simulink model "casedevsnew"  (Simulink 7.9)
settings: Solver=ode45  StartTime=0.0  StopTime=10.0  RelTol=1e-3
undefined symbols (not defined in the file or in its folder): PreNode
libraries: Post_CommonlyUsedBlocks x18, Pre_CommonlyUsedBlocks x14
settings Model: Creator=jdenil  LastModifiedBy=jdenil

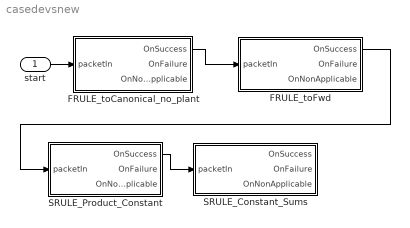
== system casedevsnew ==
  start : Inport
  FRULE_toCanonical_no_plant : Subsystem
  FRULE_toFwd : Subsystem
  SRULE_Constant_Sums : Subsystem
  SRULE_Product_Constant : Subsystem
  wires:
  start/1 -> FRULE_toCanonical_no_plant/1(packetIn)
  FRULE_toFwd/1(OnSuccess) -> SRULE_Product_Constant/1(packetIn)
  FRULE_toCanonical_no_plant/1(OnSuccess) -> FRULE_toFwd/1(packetIn)
  SRULE_Product_Constant/1(OnSuccess) -> SRULE_Constant_Sums/1(packetIn)

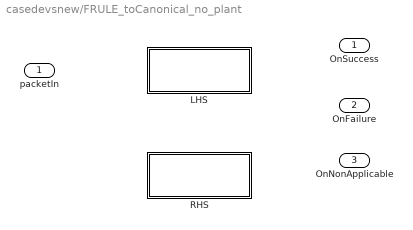
== system casedevsnew/FRULE_toCanonical_no_plant ==
  packetIn : Inport
  LHS : Subsystem  mask{Constraint=return True}
  RHS : Subsystem  mask{Action=[]}
  OnSuccess : Outport
  OnFailure : Outport  Port=2
  OnNonApplicable : Outport  Port=3

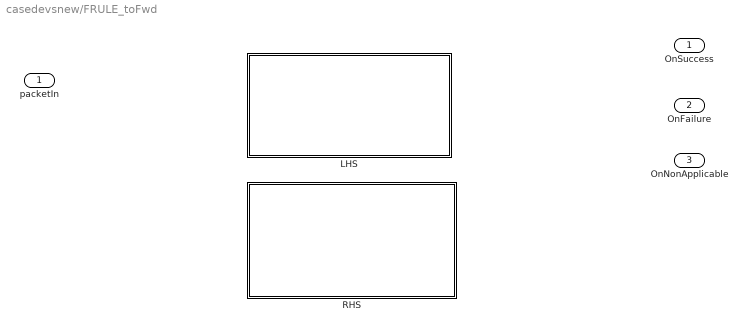
== system casedevsnew/FRULE_toFwd ==
  packetIn : Inport
  LHS : Subsystem
  RHS : Subsystem
  OnSuccess : Outport
  OnFailure : Outport  Port=2
  OnNonApplicable : Outport  Port=3

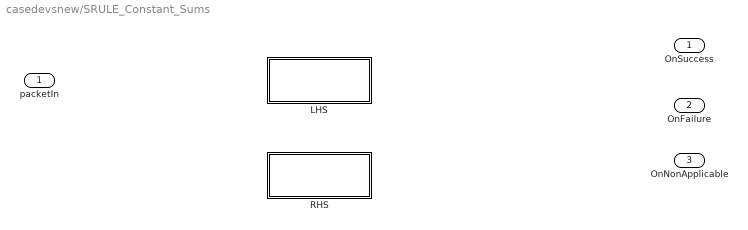
== system casedevsnew/SRULE_Constant_Sums ==
  packetIn : Inport
  LHS : Subsystem
  RHS : Subsystem
  OnSuccess : Outport
  OnFailure : Outport  Port=2
  OnNonApplicable : Outport  Port=3

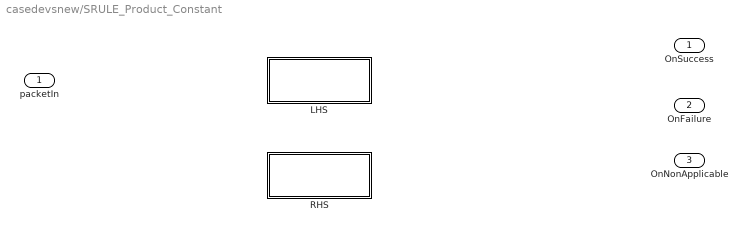
== system casedevsnew/SRULE_Product_Constant ==
  packetIn : Inport
  LHS : Subsystem
  RHS : Subsystem
  OnSuccess : Outport
  OnFailure : Outport  Port=2
  OnNonApplicable : Outport  Port=3

== system casedevsnew/FRULE_toCanonical_no_plant/LHS ==
  Atomic Subsystem : Subsystem  TreatAsAtomicUnit=on  mask{p_label=9, pre_Name=return False if 'plant' in attr_value else True, pre_Position=return True}
      settings: AttributesFormatString=%<p_label>

== system casedevsnew/FRULE_toCanonical_no_plant/RHS ==
  Atomic Subsystem : Subsystem  TreatAsAtomicUnit=on  mask{p_label=9, post_Name=return attr_value, post_Position=return attr_value}
      settings: AttributesFormatString=%<p_label>

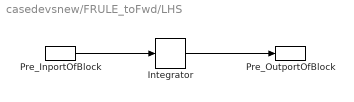
== system casedevsnew/FRULE_toFwd/LHS ==
  Integrator : Pre_CommonlyUsedBlocks/Integrator  pre_label=1  pre_initial=return True  pre_Name=return True  pre_Position=return True
      settings: AttributesFormatString=%<pre_label>
  Pre_InportOfBlock : Pre_CommonlyUsedBlocks/Pre_InportOfBlock  pre_label=0
      settings: AttributesFormatString=%<pre_label>
  Pre_OutportOfBlock : Pre_CommonlyUsedBlocks/Pre_OutportOfBlock  pre_label=2
      settings: AttributesFormatString=%<pre_label>
  wires:
  Pre_InportOfBlock/1 -> Integrator/1
  Integrator/1 -> Pre_OutportOfBlock/1

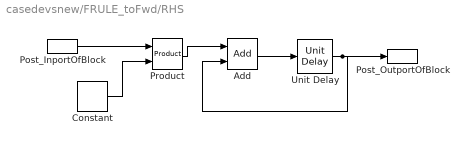
== system casedevsnew/FRULE_toFwd/RHS ==
  Add : Post_CommonlyUsedBlocks/Add  post_label=4  post_Name=return PreNode('1')['Name']+'Add'  post_Position=return PreNode('1')['Position']  post_Inputs=return '|++'
      settings: AttributesFormatString=%<post_label>
  Constant : Post_CommonlyUsedBlocks/Constant  post_label=6  post_value=return 0.001  post_Name=return PreNode('1')['Name']+'gainconst'  post_Position=return PreNode('1')['Position']
      settings: AttributesFormatString=%<post_label>
  Post_InportOfBlock : Post_CommonlyUsedBlocks/Post_InportOfBlock  post_label=0
      settings: AttributesFormatString=%<post_label>
  Post_OutportOfBlock : Post_CommonlyUsedBlocks/Post_OutportOfBlock  post_label=2
      settings: AttributesFormatString=%<post_label>
  Product : Post_CommonlyUsedBlocks/Product  post_label=3  post_Name=return PreNode('1')['Name']+'Product'  post_Position=return PreNode('1')['Position']
      settings: AttributesFormatString=%<post_label>
  Unit Delay : Post_CommonlyUsedBlocks/Unit Delay  post_label=5  post_initial=return PreNode('1')['InitialCondition']  post_Name=return PreNode('1')['Name']+'Delay'  post_Position=return PreNode('1')['Position']  post_SampleTime=return 0.001
      settings: AttributesFormatString=%<post_label>
  wires:
  Post_InportOfBlock/1 -> Product/1
  Product/1 -> Add/1
  Add/1 -> Unit Delay/1
  Unit Delay/1 -> Post_OutportOfBlock/1, Add/2
  Constant/1 -> Product/2

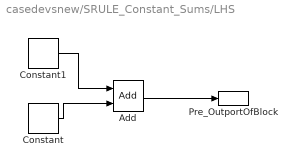
== system casedevsnew/SRULE_Constant_Sums/LHS ==
  Add : Pre_CommonlyUsedBlocks/Add  pre_label=0  pre_Name=return True  pre_Position=return True  pre_Inputs=return True
      settings: AttributesFormatString=%<pre_label>
  Constant : Pre_CommonlyUsedBlocks/Constant  pre_label=1  pre_value=return True  pre_Name=return True  pre_Position=return True
      settings: AttributesFormatString=%<pre_label>
  Constant1 : Pre_CommonlyUsedBlocks/Constant  pre_label=2  pre_value=return True  pre_Name=return True  pre_Position=return True
      settings: AttributesFormatString=%<pre_label>
  Pre_OutportOfBlock : Pre_CommonlyUsedBlocks/Pre_OutportOfBlock  pre_label=4
      settings: AttributesFormatString=%<pre_label>
  wires:
  Constant/1 -> Add/2
  Add/1 -> Pre_OutportOfBlock/1
  Constant1/1 -> Add/1

== system casedevsnew/SRULE_Constant_Sums/RHS ==
  Constant : Post_CommonlyUsedBlocks/Constant  post_label=5  post_value=return PreNode('2')['value'] + PreNode('1')['value']  post_Name=return 'folded_'+PreNode('1')['Name']+'_'+PreNode('2')['Name']  post_Position=return PreNode('0')['Position']
      settings: AttributesFormatString=%<post_label>
  Post_OutportOfBlock : Post_CommonlyUsedBlocks/Post_OutportOfBlock  post_label=4
      settings: AttributesFormatString=%<post_label>
  wires:
  Constant/1 -> Post_OutportOfBlock/1

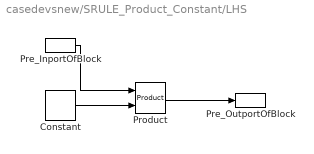
== system casedevsnew/SRULE_Product_Constant/LHS ==
  Constant : Pre_CommonlyUsedBlocks/Constant  pre_label=1  pre_value=return True  pre_Name=return True  pre_Position=return True
      settings: AttributesFormatString=%<pre_label>
  Pre_InportOfBlock : Pre_CommonlyUsedBlocks/Pre_InportOfBlock  pre_label=0
      settings: AttributesFormatString=%<pre_label>
  Pre_OutportOfBlock : Pre_CommonlyUsedBlocks/Pre_OutportOfBlock  pre_label=4
      settings: AttributesFormatString=%<pre_label>
  Product : Pre_CommonlyUsedBlocks/Product  pre_label=2  pre_Name=return True  pre_Position=return True
      settings: AttributesFormatString=%<pre_label>
  wires:
  Pre_InportOfBlock/1 -> Product/1
  Constant/1 -> Product/2
  Product/1 -> Pre_OutportOfBlock/1

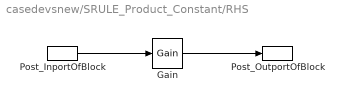
== system casedevsnew/SRULE_Product_Constant/RHS ==
  Gain : Post_CommonlyUsedBlocks/Gain  post_label=5  post_gain=return PreNode('1')['value']  post_Name=return PreNode('1')['Name']+'Gain'  post_Position=return PreNode('1')['Position']
      settings: AttributesFormatString=%<post_label>
  Post_InportOfBlock : Post_CommonlyUsedBlocks/Post_InportOfBlock  post_label=0
      settings: AttributesFormatString=%<post_label>
  Post_OutportOfBlock : Post_CommonlyUsedBlocks/Post_OutportOfBlock  post_label=4
      settings: AttributesFormatString=%<post_label>
  wires:
  Post_InportOfBlock/1 -> Gain/1
  Gain/1 -> Post_OutportOfBlock/1

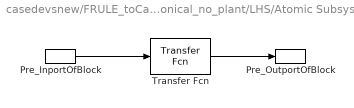
== system casedevsnew/FRULE_toCanonical_no_plant/LHS/Atomic Subsystem ==
  Pre_InportOfBlock : Pre_CommonlyUsedBlocks/Pre_InportOfBlock  pre_label=1
      settings: AttributesFormatString=%<pre_label>
  Pre_OutportOfBlock : Pre_CommonlyUsedBlocks/Pre_OutportOfBlock  pre_label=3
      settings: AttributesFormatString=%<pre_label>
  Transfer Fcn : Pre_CommonlyUsedBlocks/Transfer Fcn  pre_label=2  pre_Name=return True  pre_Position=return True  pre_Numerator=return True  pre_Denominator=return True
      settings: AttributesFormatString=%<pre_label>
  wires:
  Pre_InportOfBlock/1 -> Transfer Fcn/1
  Transfer Fcn/1 -> Pre_OutportOfBlock/1

== system casedevsnew/FRULE_toCanonical_no_plant/RHS/Atomic Subsystem ==
  Atomic Subsystem : Subsystem  TreatAsAtomicUnit=on  mask{p_label=10, post_Name=return PreNode('2')['Name']+'_unfold', post_Position=return PreNode('2')['Position']}
      settings: AttributesFormatString=%<p_label>
  Post_InportOfBlock : Post_CommonlyUsedBlocks/Post_InportOfBlock  post_label=1
      settings: AttributesFormatString=%<post_label>
  Post_OutportOfBlock : Post_CommonlyUsedBlocks/Post_OutportOfBlock  post_label=3
      settings: AttributesFormatString=%<post_label>
  wires:
  Post_InportOfBlock/1 -> Atomic Subsystem/1(Inport)
  Atomic Subsystem/1(Outport) -> Post_OutportOfBlock/1

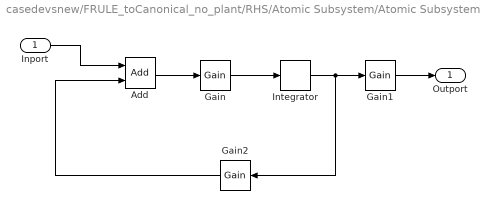
== system casedevsnew/FRULE_toCanonical_no_plant/RHS/Atomic Subsystem/Atomic Subsystem ==
  Inport : Inport  LibraryBlock=Post_CommonlyUsedBlocks/Inport  post_label=11  post_Port=return 1  post_Name=return 'In1'  post_Position=return [30,83,60,97]
      settings: AttributesFormatString=%<post_label>
  Add : Post_CommonlyUsedBlocks/Add  post_label=4  post_Name=return PreNode('2')['Name']+'_add1'  post_Position=return [135,102,165,133]  post_Inputs=return '|++'
      settings: AttributesFormatString=%<post_label>
  Gain : Post_CommonlyUsedBlocks/Gain  post_label=5  post_gain=return PreNode('2')['Denominator'][0]  post_Name=return PreNode('2')['Name']+'_Gain_D2'  post_Position=return [210,105,240,135]
      settings: AttributesFormatString=%<post_label>
  Gain1 : Post_CommonlyUsedBlocks/Gain  post_label=7  post_gain=return PreNode('2')['Numerator'][0]  post_Name=return PreNode('2')['Name']+'Gain_N_1'  post_Position=return [375,105,405,135]
      settings: AttributesFormatString=%<post_label>
  Gain2 : Post_CommonlyUsedBlocks/Gain  post_label=8  post_gain=return -PreNode('2')['Denominator'][1]  post_Name=return PreNode('2')['Name']+'_Gain_D1'  post_Position=return [230,205,260,235]
      settings: AttributesFormatString=%<post_label>
  Integrator : Post_CommonlyUsedBlocks/Integrator  post_label=6  post_initial=return 0  post_Name=return PreNode('2')['Name']+'_int'  post_Position=return [290,105,320,135]
      settings: AttributesFormatString=%<post_label>
  Outport : Outport  LibraryBlock=Post_CommonlyUsedBlocks/Outport  post_label=12  post_Port=return 1  post_Name=return 'Out1'  post_Position=return [445,113,475,127]
      settings: AttributesFormatString=%<post_label>
  wires:
  Add/1 -> Gain/1
  Gain/1 -> Integrator/1
  Integrator/1 -> Gain1/1, Gain2/1
  Gain1/1 -> Outport/1
  Gain2/1 -> Add/2
  Inport/1 -> Add/1
